simulink model "Ques7Ex6_AkankshaMurali"  (R2023b)
settings: Solver=VariableStepAuto  StartTime=0.0  StopTime=10.0  RelTol=1e-3
settings Model: Creator=akank  LastModifiedBy=akank

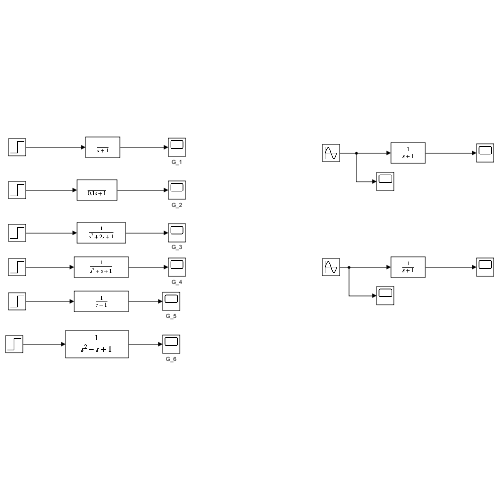
[thumbnail: Simulink's stored preview of the top-level diagram]
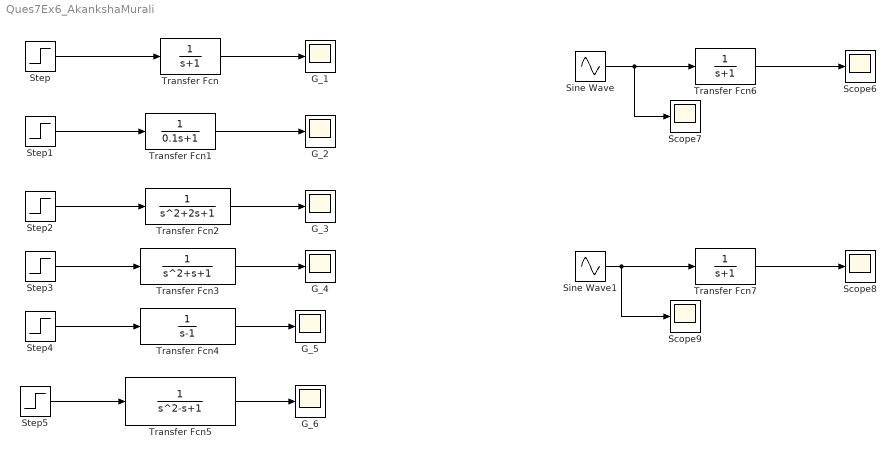
== system Ques7Ex6_AkankshaMurali ==
  G_{1..6} (6 alike) : Scope
  Scope{6..9} (4 alike) : Scope
  Sine Wave : Sin  Amplitude=0.1  SampleTime=0
  Sine Wave1 : Sin  Amplitude=20  SampleTime=0
  Step{,1..5} (6 alike) : Step  SampleTime=0
  Transfer Fcn : TransferFcn  Denominator=[1 1]
  Transfer Fcn1 : TransferFcn  Denominator=[0.1 1]
  Transfer Fcn2 : TransferFcn
  Transfer Fcn3 : TransferFcn  Denominator=[1 1 1]
  Transfer Fcn4 : TransferFcn  Denominator=[1 -1]
  Transfer Fcn5 : TransferFcn  Denominator=[1 -1 1]
  Transfer Fcn6 : TransferFcn  Denominator=[1 1]
  Transfer Fcn7 : TransferFcn  Denominator=[1 1]
  wires:
  Step5/1 -> Transfer Fcn5/1
  Transfer Fcn1/1 -> G_2/1
  Transfer Fcn2/1 -> G_3/1
  Step/1 -> Transfer Fcn/1
  Transfer Fcn4/1 -> G_5/1
  Step3/1 -> Transfer Fcn3/1
  Step4/1 -> Transfer Fcn4/1
  Step1/1 -> Transfer Fcn1/1
  Transfer Fcn/1 -> G_1/1
  Transfer Fcn3/1 -> G_4/1
  Transfer Fcn5/1 -> G_6/1
  Step2/1 -> Transfer Fcn2/1
  Sine Wave1/1 -> Transfer Fcn7/1, Scope9/1
  Sine Wave/1 -> Scope7/1, Transfer Fcn6/1
  Transfer Fcn6/1 -> Scope6/1
  Transfer Fcn7/1 -> Scope8/1
